simulink model "lookout"  (R2021a)
settings: Solver=VariableStepAuto  StartTime=0.0  StopTime=10.0  RelTol=1e-3
values from neighbouring files (symbols this model uses):
  RAD = deg2rad(A(:,2))    [init.m]    (also in init_notebook.m; rownanie_ruchu.m)
  X = A(:,1) / 1000    [init.m]    (also in init_notebook.m; rownanie_ruchu.m = A(:,1))
libraries: simulink_extras x1
settings Model: Creator=micha  LastModifiedBy=micha

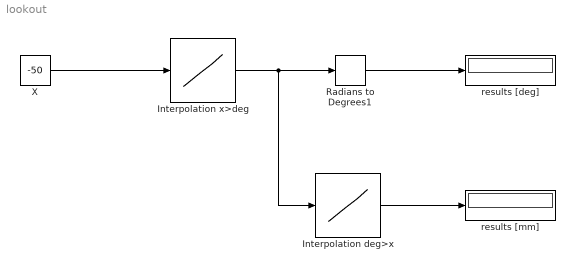
== system lookout ==
  Interpolation deg>x : Lookup_n-D  NumberOfTableDimensions=1  BreakpointsForDimension1=RAD  Table=X  InternalRulePriority=Speed  RndMeth=Simplest  InputSameDT=on
  Interpolation x>deg : Lookup_n-D  NumberOfTableDimensions=1  BreakpointsForDimension1=X  Table=RAD  InternalRulePriority=Speed  RndMeth=Simplest  InputSameDT=on
  Radians to Degrees1 : simulink_extras/Transformations/Radians to Degrees
  X : Constant  Value=-50
  results [deg] : Display
  results [mm] : Display
  wires:
  X/1 -> Interpolation x>deg/1
  Interpolation x>deg/1 -> Radians to Degrees1/1, Interpolation deg>x/1
  Radians to Degrees1/1 -> results [deg]/1
  Interpolation deg>x/1 -> results [mm]/1
